simulink model "Drone_BBall_Developer"  (R2020a)
settings: Solver=FixedStepAuto  StartTime=0.0  StopTime=60  FixedStep=.001  RelTol=1e-3
values from neighbouring files (symbols this model uses):
  b = .25*m    (= 0.25)    [Run_Match.m]
  b_ball = .02*m_ball    (= 0.01)    [Run_Match.m]
  b_F_hook = 100    [Run_Match.m]
  b_F_hoop = m_ball * 50    (= 25)    [Run_Match.m]
  b_F_R = m * 20    (= 20)    [Run_Match.m]
  b_F_R_ball = m_ball * 10    (= 5)    [Run_Match.m]
  b_F_R_hook = m_hook * 100    (= 10)    [Run_Match.m]
  B_hook = r_hook^2*6*m_ball*g    (= 0.2943)    [Run_Match.m]
  b_hook = 0.05*m_hook    (= 0.005)    [Run_Match.m]
  b_tether = 1    [Run_Match.m]
  b_th = .1*J    (= 0.0192708333333)    [Run_Match.m]
  b_th_ball = .05*J_ball    (= 0.0009)    [Run_Match.m]
  b_x_net = 80*m_ball*g    (= 392.4)    [Run_Match.m]
  b_y_net = .4*m_ball*g    (= 1.962)    [Run_Match.m]
  drone = struct([])    [Run_Match.m]    (also in animate_drone_bball.m = [-r+w -r-w -r -r r r r+w r-w;             h    h  h  0 0 h  )
  g = 9.81    [Run_Match.m]
  J = 1/4*m*r^2 + 1/12*m*(2*(r+r_M_R))^2    (= 0.192708333333)    [Run_Match.m]
  J_ball = 2/5*m_ball*r_ball^2    (= 0.018)    [Run_Match.m]
  k_f = 4    [Run_Match.m]
  k_F_hook = 10000    [Run_Match.m]
  k_F_hoop = m_ball * 5000    (= 2500)    [Run_Match.m]
  k_F_R = m * 10000    (= 10000)    [Run_Match.m]
  k_F_R_ball = m_ball * 10000    (= 5000)    [Run_Match.m]
  k_F_R_hook = m_hook * 10000    (= 1000)    [Run_Match.m]
  k_tether = 40    [Run_Match.m]
  k_x_net = 200*m_ball*g    (= 981)    [Run_Match.m]
  k_y_net = .5*m_ball*g    (= 2.4525)    [Run_Match.m]
  L_tether = 1.0    (= 1)    [Run_Match.m]
  m = 1    [Run_Match.m]
  m_ball = .5    (= 0.5)    [Run_Match.m]
  m_hook = 0.1*m    (= 0.1)    [Run_Match.m]
  mu_f = .2    (= 0.2)    [Run_Match.m]
  mu_f_gnd = 0.5    [Run_Match.m]
  p_0 = [-5; 5]    [Run_Match.m]
  p_ball_0 = [0; r_ball]    [Run_Match.m]
  p_ball_dot_0 = [0; 12]    [Run_Match.m]
  p_emp = [0; -.4]    [Run_Match.m]
  p_emp_dot = [0; -5]    [Run_Match.m]
  p_hoop = [7.5 8; 8.5 8; -8.5 8; -7.5 8]'    [Run_Match.m]
  p_tether = [0; -0.259]    [Run_Match.m]
  r = 0.5    [Run_Match.m]    (also in animate_drone_bball.m = 0.475)
  r_ball = .3    (= 0.3)    [Run_Match.m]
  r_hook = 0.1    [Run_Match.m]
  r_M_R = 0.25*r    (= 0.125)    [Run_Match.m]
  T_0 = m*g    (= 9.81)    [Run_Match.m]
  T_max = 4*m*g    (= 39.24)    [Run_Match.m]
  T_tau = 0.1    [Run_Match.m]
undefined symbols (not defined in the file or in its folder): clock, M_max, sigbuilder_block, T_aux
libraries: dspswit3 x22, simulink x17, simulink_extras x3, dspmathops x2
(part 2 of 5)

== system Drone_BBall_Developer/Drone 1 Controller/Quadcopter Dynamical Controller ==
  note: Maps the desired net thrust and
      | net moment to the corresponding
      | desired left and right rotor thrust.
  note: Measures the closest
      | angle difference, which
      | may require adding or
      | subtracting 360 degrees.
  note: The upper and lower saturation limits
      | in the X-Axis PID controller limits the
      | maximum desired angle theta to keep
      | the quadcopter upright during flight.
  note: The upper saturation limit in the
      | Y-Axis PID controller leaves some
      | room to impart a moment, even
      | when maximum thrust is desired.
  note: You will almost certainly want the compensator
      | enabled, but temporarily turning it off can be
      | useful during the design process.
  note: By adding an external theta_d to the output
      | of the X-Axis controller, the quadcopter can
      | be made to rotate (e.g., to aim the EMP). I find
      | it works pretty well to implement quick flips this
      | way, and to just fire the EMP whenever the
      |  quadcopter is pointing in the right direction.
  note: Pitch Controller
  note: Y-Axis Controller
  note: X-Axis Controller
  X : Inport
  X_d : Inport  Port=2
  Bypass : ManualSwitch  CurrentSetting=0
  Deg2Rad : Gain  Gain=pi/180
  Demux3 : Demux  Outputs=6
  Demux4 : Demux  Outputs=6
  Diff btwn Angles : Subsystem
  Mux : Mux  Inputs=6
  "Pitch Compensator " : TransferFcn  Numerator=[2 6]  Denominator=[1 10]
  Pitch PID : simulink/Continuous/PID Controller  Controller=PID  Form=Parallel  TimeDomain=Continuous-time  UseExternalTs=off  SampleTime=-1  IntegratorMethod=Forward Euler  FilterMethod=Forward Euler  ControllerParametersSource=internal  P=8  I=0  D=1  UseFilter=on  N=100  TunerSelectOption=Transfer Function Based (PID Tuner App)  InitialConditionSource=internal  InitialConditionForIntegrator=0  InitialConditionForFilter=0  DifferentiatorICPrevScaledInput=0  ExternalReset=none  TrackingMode=off  Kt=1  LimitOutput=off  UpperSaturationLimit=M_max  LowerSaturationLimit=-M_max  LinearizeAsGain=on  AntiWindupMode=none  Kb=1  POutMin=[]  POutMax=[]  IOutMin=[]  IOutMax=[]  DOutMin=[]  DOutMax=[]  NOutMin=[]  NOutMax=[]  SumOutMin=[]  SumOutMax=[]  SaturationOutMin=[]  SaturationOutMax=[]  PParamMin=[]  PParamMax=[]  IParamMin=[]  IParamMax=[]  DParamMin=[]  DParamMax=[]  NParamMin=[]  NParamMax=[]  KbParamMin=[]  KbParamMax=[]  KtParamMin=[]  KtParamMax=[]  KbOutMin=[]  KbOutMax=[]  KtOutMin=[]  KtOutMax=[]  IntegratorOutMin=[]  IntegratorOutMax=[]  FilterOutMin=[]  FilterOutMax=[]  SumI1OutMin=[]  SumI1OutMax=[]  SumI2OutMin=[]  SumI2OutMax=[]  SumI3OutMin=[]  SumI3OutMax=[]  SumI4OutMin=[]  SumI4OutMax=[]  SumDOutMin=[]  SumDOutMax=[]  DifferentiatorOutMin=[]  DifferentiatorOutMax=[]  FilterDiffOutCoefMin=[]  FilterDiffOutCoefMax=[]  ReciprocalOutMin=[]  ReciprocalOutMax=[]  SumDenOutMin=[]  SumDenOutMax=[]  SumNumOutMin=[]  SumNumOutMax=[]  DivideOutMin=[]  DivideOutMax=[]  UdiffTsProdOutMin=[]  UdiffTsProdOutMax=[]  NTsProdOutMin=[]  NTsProdOutMax=[]  UintegralTsProdOutMin=[]  UintegralTsProdOutMax=[]  UngainTsProdOutMin=[]  UngainTsProdOutMax=[]  IntegratorContinuousStateAttributes=''  IntegratorStateMustResolveToSignalObject=off  IntegratorRTWStateStorageClass=Auto  FilterContinuousStateAttributes=''  FilterStateMustResolveToSignalObject=off  FilterRTWStateStorageClass=Auto  ParallelPVariant=InternalParameters  IdealPVariant=Disabled  IVariant=InternalParameters  DVariant=InternalParameters  IntegratorVariant=Continuous  SatVariant=Disabled  AWVariant=Passthrough  PCopyVariant=Disabled  TRVariant=Disabled  FdbkBlocksVariant=Forward  IdealPFdbkVariant=Disabled  SatFdbkVariant=Disabled  DerivativeFilterVariant=ContFilter  NVariant=InternalParameters  NCopyVariant=Disabled  FilterICVariant=InternalICsFilter  IntegratorICVariant=InternalICs  ExternalResetVariant=Disabled  TRSumVariant=Passthrough  SumFdbkVariant=Disabled  SumVariant=Sum_PID  TsampFilterVariant=InternalTs  TsampNgainVariant=Passthrough  TsampIntegralVariant=Passthrough
  Sum : Sum  Inputs=|++
  Sum1 : Sum  Inputs=-|+
  Sum2 : Sum  Inputs=-|+
  Terminator1 : Terminator
  Terminator2 : Terminator
  Terminator7 : Terminator
  Thurst Mapping : Subsystem
  Wrap Angle : Subsystem
  X_Axis PID : simulink/Continuous/PID Controller  Controller=PID  Form=Parallel  TimeDomain=Continuous-time  UseExternalTs=off  SampleTime=-1  IntegratorMethod=Forward Euler  FilterMethod=Forward Euler  ControllerParametersSource=internal  P=8  I=2  D=4  UseFilter=on  N=100  TunerSelectOption=Transfer Function Based (PID Tuner App)  InitialConditionSource=internal  InitialConditionForIntegrator=0  InitialConditionForFilter=0  DifferentiatorICPrevScaledInput=0  ExternalReset=none  TrackingMode=off  Kt=1  LimitOutput=on  UpperSaturationLimit=60  LowerSaturationLimit=-60  LinearizeAsGain=on  AntiWindupMode=clamping  Kb=1  POutMin=[]  POutMax=[]  IOutMin=[]  IOutMax=[]  DOutMin=[]  DOutMax=[]  NOutMin=[]  NOutMax=[]  SumOutMin=[]  SumOutMax=[]  SaturationOutMin=[]  SaturationOutMax=[]  PParamMin=[]  PParamMax=[]  IParamMin=[]  IParamMax=[]  DParamMin=[]  DParamMax=[]  NParamMin=[]  NParamMax=[]  KbParamMin=[]  KbParamMax=[]  KtParamMin=[]  KtParamMax=[]  KbOutMin=[]  KbOutMax=[]  KtOutMin=[]  KtOutMax=[]  IntegratorOutMin=[]  IntegratorOutMax=[]  FilterOutMin=[]  FilterOutMax=[]  SumI1OutMin=[]  SumI1OutMax=[]  SumI2OutMin=[]  SumI2OutMax=[]  SumI3OutMin=[]  SumI3OutMax=[]  SumI4OutMin=[]  SumI4OutMax=[]  SumDOutMin=[]  SumDOutMax=[]  DifferentiatorOutMin=[]  DifferentiatorOutMax=[]  FilterDiffOutCoefMin=[]  FilterDiffOutCoefMax=[]  ReciprocalOutMin=[]  ReciprocalOutMax=[]  SumDenOutMin=[]  SumDenOutMax=[]  SumNumOutMin=[]  SumNumOutMax=[]  DivideOutMin=[]  DivideOutMax=[]  UdiffTsProdOutMin=[]  UdiffTsProdOutMax=[]  NTsProdOutMin=[]  NTsProdOutMax=[]  UintegralTsProdOutMin=[]  UintegralTsProdOutMax=[]  UngainTsProdOutMin=[]  UngainTsProdOutMax=[]  IntegratorContinuousStateAttributes=''  IntegratorStateMustResolveToSignalObject=off  IntegratorRTWStateStorageClass=Auto  FilterContinuousStateAttributes=''  FilterStateMustResolveToSignalObject=off  FilterRTWStateStorageClass=Auto  ParallelPVariant=InternalParameters  IdealPVariant=Disabled  IVariant=InternalParameters  DVariant=InternalParameters  IntegratorVariant=Continuous  SatVariant=Enabled  AWVariant=ContClampingParallel  PCopyVariant=Disabled  TRVariant=Disabled  FdbkBlocksVariant=Forward  IdealPFdbkVariant=Disabled  SatFdbkVariant=Disabled  DerivativeFilterVariant=ContFilter  NVariant=InternalParameters  NCopyVariant=Disabled  FilterICVariant=InternalICsFilter  IntegratorICVariant=InternalICs  ExternalResetVariant=Disabled  TRSumVariant=Passthrough  SumFdbkVariant=Disabled  SumVariant=Sum_PID  TsampFilterVariant=InternalTs  TsampNgainVariant=Passthrough  TsampIntegralVariant=Passthrough
  Y_Axis PID : simulink/Continuous/PID Controller  Controller=PID  Form=Parallel  TimeDomain=Continuous-time  UseExternalTs=off  SampleTime=-1  IntegratorMethod=Forward Euler  FilterMethod=Forward Euler  ControllerParametersSource=internal  P=36.8701654473811  I=116.471336399404  D=12.6703199505361  UseFilter=on  N=100  TunerSelectOption=Transfer Function Based (PID Tuner App)  InitialConditionSource=internal  InitialConditionForIntegrator=m*g  InitialConditionForFilter=0  DifferentiatorICPrevScaledInput=0  ExternalReset=none  TrackingMode=off  Kt=1  LimitOutput=on  UpperSaturationLimit=T_max - 2*T_aux  LowerSaturationLimit=0  LinearizeAsGain=on  AntiWindupMode=clamping  Kb=1  POutMin=[]  POutMax=[]  IOutMin=[]  IOutMax=[]  DOutMin=[]  DOutMax=[]  NOutMin=[]  NOutMax=[]  SumOutMin=[]  SumOutMax=[]  SaturationOutMin=[]  SaturationOutMax=[]  PParamMin=[]  PParamMax=[]  IParamMin=[]  IParamMax=[]  DParamMin=[]  DParamMax=[]  NParamMin=[]  NParamMax=[]  KbParamMin=[]  KbParamMax=[]  KtParamMin=[]  KtParamMax=[]  KbOutMin=[]  KbOutMax=[]  KtOutMin=[]  KtOutMax=[]  IntegratorOutMin=[]  IntegratorOutMax=[]  FilterOutMin=[]  FilterOutMax=[]  SumI1OutMin=[]  SumI1OutMax=[]  SumI2OutMin=[]  SumI2OutMax=[]  SumI3OutMin=[]  SumI3OutMax=[]  SumI4OutMin=[]  SumI4OutMax=[]  SumDOutMin=[]  SumDOutMax=[]  DifferentiatorOutMin=[]  DifferentiatorOutMax=[]  FilterDiffOutCoefMin=[]  FilterDiffOutCoefMax=[]  ReciprocalOutMin=[]  ReciprocalOutMax=[]  SumDenOutMin=[]  SumDenOutMax=[]  SumNumOutMin=[]  SumNumOutMax=[]  DivideOutMin=[]  DivideOutMax=[]  UdiffTsProdOutMin=[]  UdiffTsProdOutMax=[]  NTsProdOutMin=[]  NTsProdOutMax=[]  UintegralTsProdOutMin=[]  UintegralTsProdOutMax=[]  UngainTsProdOutMin=[]  UngainTsProdOutMax=[]  IntegratorContinuousStateAttributes=''  IntegratorStateMustResolveToSignalObject=off  IntegratorRTWStateStorageClass=Auto  FilterContinuousStateAttributes=''  FilterStateMustResolveToSignalObject=off  FilterRTWStateStorageClass=Auto  ParallelPVariant=InternalParameters  IdealPVariant=Disabled  IVariant=InternalParameters  DVariant=InternalParameters  IntegratorVariant=Continuous  SatVariant=Enabled  AWVariant=ContClampingParallel  PCopyVariant=Disabled  TRVariant=Disabled  FdbkBlocksVariant=Forward  IdealPFdbkVariant=Disabled  SatFdbkVariant=Disabled  DerivativeFilterVariant=ContFilter  NVariant=InternalParameters  NCopyVariant=Disabled  FilterICVariant=InternalICsFilter  IntegratorICVariant=InternalICs  ExternalResetVariant=Disabled  TRSumVariant=Passthrough  SumFdbkVariant=Disabled  SumVariant=Sum_PID  TsampFilterVariant=InternalTs  TsampNgainVariant=Passthrough  TsampIntegralVariant=Passthrough
  T_L_d : Outport  VectorParamsAs1DForOutWhenUnconnected=off
  T_R_d : Outport  Port=2  VectorParamsAs1DForOutWhenUnconnected=off
  X_d_adj : Outport  Port=3  VectorParamsAs1DForOutWhenUnconnected=off
  wires:
  Thurst Mapping/2(T_R_d) -> T_R_d/1
  X_Axis PID/1 -> Deg2Rad/1
  "Pitch Compensator "/1 -> Bypass/2
  Bypass/1 -> Pitch PID/1
  Pitch PID/1 -> Thurst Mapping/1(M_d)
  Thurst Mapping/1(T_L_d) -> T_L_d/1
  Y_Axis PID/1 -> Thurst Mapping/2(T_d)
  Demux3/6 -> Mux/6
  Demux4/6 -> Terminator7/1
  Demux4/5 -> Diff btwn Angles/1(theta)  "theta"
  X_d/1 -> Demux3/1
  Demux4/1 -> Sum1/1  "x"
  Demux3/1 -> Mux/1, Sum1/2  "x_d"
  Demux4/3 -> Sum2/1  "y"
  Demux3/3 -> Sum2/2, Mux/3  "y_d"
  Demux3/2 -> Mux/2
  Demux3/4 -> Mux/4
  Demux3/5 -> Sum/2
  Sum/1 -> Wrap Angle/1(raw), Diff btwn Angles/2(theta_d)  "theta_d"
  X/1 -> Demux4/1
  Mux/1 -> X_d_adj/1
  Diff btwn Angles/1(e) -> Bypass/1, "Pitch Compensator "/1
  Wrap Angle/1(wrap) -> Mux/5
  Demux4/2 -> Terminator1/1
  Demux4/4 -> Terminator2/1
  Sum2/1 -> Y_Axis PID/1
  Sum1/1 -> X_Axis PID/1
  Deg2Rad/1 -> Sum/1

== system Drone_BBall_Developer/Drone 1 Controller/Quadcopter Dynamical Controller (Arena Frame) ==
  note: Maps the desired net thrust and
      | net moment to the corresponding
      | desired left and right rotor thrust.
  note: Measures the closest
      | angle difference, which
      | may require adding or
      | subtracting 360 degrees.
  note: The upper and lower saturation limits
      | in the X-Axis PID controller limits the
      | maximum desired angle theta to keep
      | the quadcopter upright during flight.
  note: The upper saturation limit in the
      | Y-Axis PID controller leaves some
      | room to impart a moment, even
      | when maximum thrust is desired.
  note: You will almost certainly want the compensator
      | enabled, but temporarily turning it off can be
      | useful during the design process.
  note: By adding an external theta_d to the output
      | of the X-Axis controller, the quadcopter can
      | be made to rotate (e.g., to aim the EMP). I find
      | it works pretty well to implement quick flips this
      | way, and to just fire the EMP whenever the
      |  quadcopter is pointing in the right direction.
  note: Pitch Controller
  note: Y-Axis Controller
  note: X-Axis Controller
  X : Inport
  X_d : Inport  Port=2
  Bypass : ManualSwitch
  Deg2Rad : Gain  Gain=pi/180
  Demux3 : Demux  Outputs=6
  Demux4 : Demux  Outputs=6
  Diff btwn Angles : Subsystem
  Mux : Mux  Inputs=6
  "Pitch Compensator " : TransferFcn  Numerator=[2 6]  Denominator=[1 10]
  Pitch PID : simulink/Continuous/PID Controller  Controller=PID  Form=Parallel  TimeDomain=Continuous-time  UseExternalTs=off  SampleTime=-1  IntegratorMethod=Forward Euler  FilterMethod=Forward Euler  ControllerParametersSource=internal  P=8  I=0  D=1  UseFilter=on  N=100  TunerSelectOption=Transfer Function Based (PID Tuner App)  InitialConditionSource=internal  InitialConditionForIntegrator=0  InitialConditionForFilter=0  DifferentiatorICPrevScaledInput=0  ExternalReset=none  TrackingMode=off  Kt=1  LimitOutput=off  UpperSaturationLimit=M_max  LowerSaturationLimit=-M_max  LinearizeAsGain=on  AntiWindupMode=none  Kb=1  POutMin=[]  POutMax=[]  IOutMin=[]  IOutMax=[]  DOutMin=[]  DOutMax=[]  NOutMin=[]  NOutMax=[]  SumOutMin=[]  SumOutMax=[]  SaturationOutMin=[]  SaturationOutMax=[]  PParamMin=[]  PParamMax=[]  IParamMin=[]  IParamMax=[]  DParamMin=[]  DParamMax=[]  NParamMin=[]  NParamMax=[]  KbParamMin=[]  KbParamMax=[]  KtParamMin=[]  KtParamMax=[]  KbOutMin=[]  KbOutMax=[]  KtOutMin=[]  KtOutMax=[]  IntegratorOutMin=[]  IntegratorOutMax=[]  FilterOutMin=[]  FilterOutMax=[]  SumI1OutMin=[]  SumI1OutMax=[]  SumI2OutMin=[]  SumI2OutMax=[]  SumI3OutMin=[]  SumI3OutMax=[]  SumI4OutMin=[]  SumI4OutMax=[]  SumDOutMin=[]  SumDOutMax=[]  DifferentiatorOutMin=[]  DifferentiatorOutMax=[]  FilterDiffOutCoefMin=[]  FilterDiffOutCoefMax=[]  ReciprocalOutMin=[]  ReciprocalOutMax=[]  SumDenOutMin=[]  SumDenOutMax=[]  SumNumOutMin=[]  SumNumOutMax=[]  DivideOutMin=[]  DivideOutMax=[]  UdiffTsProdOutMin=[]  UdiffTsProdOutMax=[]  NTsProdOutMin=[]  NTsProdOutMax=[]  UintegralTsProdOutMin=[]  UintegralTsProdOutMax=[]  UngainTsProdOutMin=[]  UngainTsProdOutMax=[]  IntegratorContinuousStateAttributes=''  IntegratorStateMustResolveToSignalObject=off  IntegratorRTWStateStorageClass=Auto  FilterContinuousStateAttributes=''  FilterStateMustResolveToSignalObject=off  FilterRTWStateStorageClass=Auto  ParallelPVariant=InternalParameters  IdealPVariant=Disabled  IVariant=InternalParameters  DVariant=InternalParameters  IntegratorVariant=Continuous  SatVariant=Disabled  AWVariant=Passthrough  PCopyVariant=Disabled  TRVariant=Disabled  FdbkBlocksVariant=Forward  IdealPFdbkVariant=Disabled  SatFdbkVariant=Disabled  DerivativeFilterVariant=ContFilter  NVariant=InternalParameters  NCopyVariant=Disabled  FilterICVariant=InternalICsFilter  IntegratorICVariant=InternalICs  ExternalResetVariant=Disabled  TRSumVariant=Passthrough  SumFdbkVariant=Disabled  SumVariant=Sum_PID  TsampFilterVariant=InternalTs  TsampNgainVariant=Passthrough  TsampIntegralVariant=Passthrough
  Sum : Sum  Inputs=|++
  Sum1 : Sum  Inputs=-|+
  Sum2 : Sum  Inputs=-|+
  Terminator1 : Terminator
  Terminator2 : Terminator
  Terminator7 : Terminator
  Thurst Mapping : Subsystem
  Wrap Angle : Subsystem
  X_Axis PID : simulink/Continuous/PID Controller  Controller=PID  Form=Parallel  TimeDomain=Continuous-time  UseExternalTs=off  SampleTime=-1  IntegratorMethod=Forward Euler  FilterMethod=Forward Euler  ControllerParametersSource=internal  P=8  I=2  D=4  UseFilter=on  N=100  TunerSelectOption=Transfer Function Based (PID Tuner App)  InitialConditionSource=internal  InitialConditionForIntegrator=0  InitialConditionForFilter=0  DifferentiatorICPrevScaledInput=0  ExternalReset=none  TrackingMode=off  Kt=1  LimitOutput=on  UpperSaturationLimit=60  LowerSaturationLimit=-60  LinearizeAsGain=on  AntiWindupMode=clamping  Kb=1  POutMin=[]  POutMax=[]  IOutMin=[]  IOutMax=[]  DOutMin=[]  DOutMax=[]  NOutMin=[]  NOutMax=[]  SumOutMin=[]  SumOutMax=[]  SaturationOutMin=[]  SaturationOutMax=[]  PParamMin=[]  PParamMax=[]  IParamMin=[]  IParamMax=[]  DParamMin=[]  DParamMax=[]  NParamMin=[]  NParamMax=[]  KbParamMin=[]  KbParamMax=[]  KtParamMin=[]  KtParamMax=[]  KbOutMin=[]  KbOutMax=[]  KtOutMin=[]  KtOutMax=[]  IntegratorOutMin=[]  IntegratorOutMax=[]  FilterOutMin=[]  FilterOutMax=[]  SumI1OutMin=[]  SumI1OutMax=[]  SumI2OutMin=[]  SumI2OutMax=[]  SumI3OutMin=[]  SumI3OutMax=[]  SumI4OutMin=[]  SumI4OutMax=[]  SumDOutMin=[]  SumDOutMax=[]  DifferentiatorOutMin=[]  DifferentiatorOutMax=[]  FilterDiffOutCoefMin=[]  FilterDiffOutCoefMax=[]  ReciprocalOutMin=[]  ReciprocalOutMax=[]  SumDenOutMin=[]  SumDenOutMax=[]  SumNumOutMin=[]  SumNumOutMax=[]  DivideOutMin=[]  DivideOutMax=[]  UdiffTsProdOutMin=[]  UdiffTsProdOutMax=[]  NTsProdOutMin=[]  NTsProdOutMax=[]  UintegralTsProdOutMin=[]  UintegralTsProdOutMax=[]  UngainTsProdOutMin=[]  UngainTsProdOutMax=[]  IntegratorContinuousStateAttributes=''  IntegratorStateMustResolveToSignalObject=off  IntegratorRTWStateStorageClass=Auto  FilterContinuousStateAttributes=''  FilterStateMustResolveToSignalObject=off  FilterRTWStateStorageClass=Auto  ParallelPVariant=InternalParameters  IdealPVariant=Disabled  IVariant=InternalParameters  DVariant=InternalParameters  IntegratorVariant=Continuous  SatVariant=Enabled  AWVariant=ContClampingParallel  PCopyVariant=Disabled  TRVariant=Disabled  FdbkBlocksVariant=Forward  IdealPFdbkVariant=Disabled  SatFdbkVariant=Disabled  DerivativeFilterVariant=ContFilter  NVariant=InternalParameters  NCopyVariant=Disabled  FilterICVariant=InternalICsFilter  IntegratorICVariant=InternalICs  ExternalResetVariant=Disabled  TRSumVariant=Passthrough  SumFdbkVariant=Disabled  SumVariant=Sum_PID  TsampFilterVariant=InternalTs  TsampNgainVariant=Passthrough  TsampIntegralVariant=Passthrough
  Y_Axis PID : simulink/Continuous/PID Controller  Controller=PID  Form=Parallel  TimeDomain=Continuous-time  UseExternalTs=off  SampleTime=-1  IntegratorMethod=Forward Euler  FilterMethod=Forward Euler  ControllerParametersSource=internal  P=5  I=4  D=1  UseFilter=on  N=100  TunerSelectOption=Transfer Function Based (PID Tuner App)  InitialConditionSource=internal  InitialConditionForIntegrator=m*g  InitialConditionForFilter=0  DifferentiatorICPrevScaledInput=0  ExternalReset=none  TrackingMode=off  Kt=1  LimitOutput=on  UpperSaturationLimit=T_max - 0.2  LowerSaturationLimit=0  LinearizeAsGain=on  AntiWindupMode=clamping  Kb=1  POutMin=[]  POutMax=[]  IOutMin=[]  IOutMax=[]  DOutMin=[]  DOutMax=[]  NOutMin=[]  NOutMax=[]  SumOutMin=[]  SumOutMax=[]  SaturationOutMin=[]  SaturationOutMax=[]  PParamMin=[]  PParamMax=[]  IParamMin=[]  IParamMax=[]  DParamMin=[]  DParamMax=[]  NParamMin=[]  NParamMax=[]  KbParamMin=[]  KbParamMax=[]  KtParamMin=[]  KtParamMax=[]  KbOutMin=[]  KbOutMax=[]  KtOutMin=[]  KtOutMax=[]  IntegratorOutMin=[]  IntegratorOutMax=[]  FilterOutMin=[]  FilterOutMax=[]  SumI1OutMin=[]  SumI1OutMax=[]  SumI2OutMin=[]  SumI2OutMax=[]  SumI3OutMin=[]  SumI3OutMax=[]  SumI4OutMin=[]  SumI4OutMax=[]  SumDOutMin=[]  SumDOutMax=[]  DifferentiatorOutMin=[]  DifferentiatorOutMax=[]  FilterDiffOutCoefMin=[]  FilterDiffOutCoefMax=[]  ReciprocalOutMin=[]  ReciprocalOutMax=[]  SumDenOutMin=[]  SumDenOutMax=[]  SumNumOutMin=[]  SumNumOutMax=[]  DivideOutMin=[]  DivideOutMax=[]  UdiffTsProdOutMin=[]  UdiffTsProdOutMax=[]  NTsProdOutMin=[]  NTsProdOutMax=[]  UintegralTsProdOutMin=[]  UintegralTsProdOutMax=[]  UngainTsProdOutMin=[]  UngainTsProdOutMax=[]  IntegratorContinuousStateAttributes=''  IntegratorStateMustResolveToSignalObject=off  IntegratorRTWStateStorageClass=Auto  FilterContinuousStateAttributes=''  FilterStateMustResolveToSignalObject=off  FilterRTWStateStorageClass=Auto  ParallelPVariant=InternalParameters  IdealPVariant=Disabled  IVariant=InternalParameters  DVariant=InternalParameters  IntegratorVariant=Continuous  SatVariant=Enabled  AWVariant=ContClampingParallel  PCopyVariant=Disabled  TRVariant=Disabled  FdbkBlocksVariant=Forward  IdealPFdbkVariant=Disabled  SatFdbkVariant=Disabled  DerivativeFilterVariant=ContFilter  NVariant=InternalParameters  NCopyVariant=Disabled  FilterICVariant=InternalICsFilter  IntegratorICVariant=InternalICs  ExternalResetVariant=Disabled  TRSumVariant=Passthrough  SumFdbkVariant=Disabled  SumVariant=Sum_PID  TsampFilterVariant=InternalTs  TsampNgainVariant=Passthrough  TsampIntegralVariant=Passthrough
  T_L_d : Outport  VectorParamsAs1DForOutWhenUnconnected=off
  T_R_d : Outport  Port=2  VectorParamsAs1DForOutWhenUnconnected=off
  X_d_adj : Outport  Port=3  VectorParamsAs1DForOutWhenUnconnected=off
  wires:
  Thurst Mapping/2(T_R_d) -> T_R_d/1
  X_Axis PID/1 -> Deg2Rad/1
  "Pitch Compensator "/1 -> Bypass/2
  Bypass/1 -> Pitch PID/1
  Pitch PID/1 -> Thurst Mapping/1(M_d)
  Thurst Mapping/1(T_L_d) -> T_L_d/1
  Y_Axis PID/1 -> Thurst Mapping/2(T_d)
  Demux3/6 -> Mux/6
  Demux4/6 -> Terminator7/1
  Demux4/5 -> Diff btwn Angles/1(theta)  "theta"
  X_d/1 -> Demux3/1
  Demux4/1 -> Sum1/1  "x"
  Demux3/1 -> Mux/1, Sum1/2  "x_d"
  Demux4/3 -> Sum2/1  "y"
  Demux3/3 -> Sum2/2, Mux/3  "y_d"
  Demux3/2 -> Mux/2
  Demux3/4 -> Mux/4
  Demux3/5 -> Sum/2
  Sum/1 -> Wrap Angle/1(raw), Diff btwn Angles/2(theta_d)  "theta_d"
  X/1 -> Demux4/1
  Mux/1 -> X_d_adj/1
  Diff btwn Angles/1(e) -> Bypass/1, "Pitch Compensator "/1
  Wrap Angle/1(wrap) -> Mux/5
  Demux4/2 -> Terminator1/1
  Demux4/4 -> Terminator2/1
  Sum2/1 -> Y_Axis PID/1
  Sum1/1 -> X_Axis PID/1
  Deg2Rad/1 -> Sum/1

== system Drone_BBall_Developer/Drone 1 Controller/Quadcopter Dynamical Controller (Drone Frame) ==
  note: Maps the desired net thrust and
      | net moment to the corresponding
      | desired left and right rotor thrust.
  note: Measures the closest
      | angle difference, which
      | may require adding or
      | subtracting 360 degrees.
  note: These subsystems rotate the error
      | signal, and its derivative, so that they
      | are reported in the quadcopter's
      | frame of reference. This prevents its
      | rotation from affecting the derivative
      | error terms used by the PID controllers.
  note: The upper and lower saturation limits
      | in the X-Axis PID controller limits the
      | maximum desired angle theta to keep
      | the quadcopter upright during flight.
      |
      | (I had to build custom anti-windup
      | PID controllers for X- and Y-axis to
      | separate e and e_dot inputs.)
  note: The upper saturation limit in the
      | Y-Axis PID controller leaves some
      | room to impart a moment, even
      | when maximum thrust is desired.
  note: You will almost certainly want the compensator
      | enabled, but temporarily turning it off can be
      | useful during the design process.
  note: By adding an external theta_d to the output of the X-Axis controller,
      | the quadcopter can be made to rotate (e.g., to aim the EMP). I find
      | it works pretty well to implement quick flips this way, and to just fire
      | the EMP whenever the quadcopter is pointing in the right direction.
  note: Pitch Controller
  note: Y-Axis Controller
  note: X-Axis Controller
  note: Rotate Error Signals
  X : Inport
  X_d : Inport  Port=2
  Bypass : ManualSwitch  CurrentSetting=0
  Demux : Demux  Outputs=2
  Demux1 : Demux  Outputs=2
  Demux3 : Demux  Outputs=6
  Demux4 : Demux  Outputs=6
  Diff btwn Angles : Subsystem
  Mux : Mux  Inputs=6
  Mux1 : Mux  Inputs=2
  Mux3 : Mux  Inputs=2
  "Pitch Compensator " : TransferFcn  Numerator=[2 6]  Denominator=[1 10]
  Pitch PID : simulink/Continuous/PID Controller  Controller=PID  Form=Parallel  TimeDomain=Continuous-time  UseExternalTs=off  SampleTime=-1  IntegratorMethod=Forward Euler  FilterMethod=Forward Euler  ControllerParametersSource=internal  P=8  I=0  D=1  UseFilter=on  N=100  TunerSelectOption=Transfer Function Based (PID Tuner App)  InitialConditionSource=internal  InitialConditionForIntegrator=0  InitialConditionForFilter=0  DifferentiatorICPrevScaledInput=0  ExternalReset=none  TrackingMode=off  Kt=1  LimitOutput=off  UpperSaturationLimit=M_max  LowerSaturationLimit=-M_max  LinearizeAsGain=on  AntiWindupMode=none  Kb=1  POutMin=[]  POutMax=[]  IOutMin=[]  IOutMax=[]  DOutMin=[]  DOutMax=[]  NOutMin=[]  NOutMax=[]  SumOutMin=[]  SumOutMax=[]  SaturationOutMin=[]  SaturationOutMax=[]  PParamMin=[]  PParamMax=[]  IParamMin=[]  IParamMax=[]  DParamMin=[]  DParamMax=[]  NParamMin=[]  NParamMax=[]  KbParamMin=[]  KbParamMax=[]  KtParamMin=[]  KtParamMax=[]  KbOutMin=[]  KbOutMax=[]  KtOutMin=[]  KtOutMax=[]  IntegratorOutMin=[]  IntegratorOutMax=[]  FilterOutMin=[]  FilterOutMax=[]  SumI1OutMin=[]  SumI1OutMax=[]  SumI2OutMin=[]  SumI2OutMax=[]  SumI3OutMin=[]  SumI3OutMax=[]  SumI4OutMin=[]  SumI4OutMax=[]  SumDOutMin=[]  SumDOutMax=[]  DifferentiatorOutMin=[]  DifferentiatorOutMax=[]  FilterDiffOutCoefMin=[]  FilterDiffOutCoefMax=[]  ReciprocalOutMin=[]  ReciprocalOutMax=[]  SumDenOutMin=[]  SumDenOutMax=[]  SumNumOutMin=[]  SumNumOutMax=[]  DivideOutMin=[]  DivideOutMax=[]  UdiffTsProdOutMin=[]  UdiffTsProdOutMax=[]  NTsProdOutMin=[]  NTsProdOutMax=[]  UintegralTsProdOutMin=[]  UintegralTsProdOutMax=[]  UngainTsProdOutMin=[]  UngainTsProdOutMax=[]  IntegratorContinuousStateAttributes=''  IntegratorStateMustResolveToSignalObject=off  IntegratorRTWStateStorageClass=Auto  FilterContinuousStateAttributes=''  FilterStateMustResolveToSignalObject=off  FilterRTWStateStorageClass=Auto  ParallelPVariant=InternalParameters  IdealPVariant=Disabled  IVariant=InternalParameters  DVariant=InternalParameters  IntegratorVariant=Continuous  SatVariant=Disabled  AWVariant=Passthrough  PCopyVariant=Disabled  TRVariant=Disabled  FdbkBlocksVariant=Forward  IdealPFdbkVariant=Disabled  SatFdbkVariant=Disabled  DerivativeFilterVariant=ContFilter  NVariant=InternalParameters  NCopyVariant=Disabled  FilterICVariant=InternalICsFilter  IntegratorICVariant=InternalICs  ExternalResetVariant=Disabled  TRSumVariant=Passthrough  SumFdbkVariant=Disabled  SumVariant=Sum_PID  TsampFilterVariant=InternalTs  TsampNgainVariant=Passthrough  TsampIntegralVariant=Passthrough
  Rotate e (CCW) : Subsystem
  Rotate e_dot (CCW) : Subsystem
  Sum : Sum  Inputs=|++
  Sum{1..4} (4 alike) : Sum  Inputs=-|+
  Terminator7 : Terminator
  Thurst Mapping : Subsystem
  Wrap Angle : Subsystem
  X-Axis PID : Subsystem  mask{u_max=40, K_P=8, K_I=2, K_D=4}
      mask prompts: u_max "Integration Bound (degrees)"; K_P "Proportional Gain"; K_I "Integral Gain"; K_D "Derivative Gain"
  Y-Axis PID : Subsystem  mask{u_max=T_max - 0.2, u_0=m*g, K_P=5, K_I=4, K_D=1}
      mask prompts: u_max "Integration Bound (N)"; u_0 "Initial Thrust (N)"; K_P "Proportional Gain"; K_I "Integral Gain"; K_D "Derivative Gain"
  T_L_d : Outport  VectorParamsAs1DForOutWhenUnconnected=off
  T_R_d : Outport  Port=2  VectorParamsAs1DForOutWhenUnconnected=off
  X_d_adj : Outport  Port=3  VectorParamsAs1DForOutWhenUnconnected=off
  wires:
  Thurst Mapping/2(T_R_d) -> T_R_d/1
  X-Axis PID/1(u) -> Sum/1
  "Pitch Compensator "/1 -> Bypass/2
  Bypass/1 -> Pitch PID/1
  Pitch PID/1 -> Thurst Mapping/1(M_d)
  Thurst Mapping/1(T_L_d) -> T_L_d/1
  Rotate e_dot (CCW)/1(R(theta)*p) -> Demux1/1
  Rotate e (CCW)/1(R(theta)*p) -> Demux/1
  Demux1/1 -> X-Axis PID/2(e_dot)
  Demux1/2 -> Y-Axis PID/2(e_dot)
  Y-Axis PID/1(u) -> Thurst Mapping/2(T_d)
  Demux3/6 -> Mux/6
  Demux4/6 -> Terminator7/1
  Demux4/5 -> Rotate e (CCW)/2(theta), Rotate e_dot (CCW)/2(theta), Diff btwn Angles/1(theta)  "theta"
  Mux1/1 -> Rotate e (CCW)/1(p)
  Mux3/1 -> Rotate e_dot (CCW)/1(p)
  X_d/1 -> Demux3/1
  Demux4/1 -> Sum1/1  "x"
  Demux3/1 -> Mux/1, Sum1/2  "x_d"
  Sum1/1 -> Mux1/1
  Demux4/3 -> Sum2/1  "y"
  Demux3/3 -> Mux/3, Sum2/2  "y_d"
  Demux3/2 -> Mux/2, Sum3/2
  Demux4/2 -> Sum3/1
  Sum3/1 -> Mux3/1
  Sum4/1 -> Mux3/2
  Demux4/4 -> Sum4/1
  Demux3/4 -> Mux/4, Sum4/2
  Demux3/5 -> Sum/2
  Sum/1 -> Wrap Angle/1(raw), Diff btwn Angles/2(theta_d)  "theta_d"
  X/1 -> Demux4/1
  Mux/1 -> X_d_adj/1
  Diff btwn Angles/1(e) -> Bypass/1, "Pitch Compensator "/1
  Wrap Angle/1(wrap) -> Mux/5
  Demux/1 -> X-Axis PID/1(e)
  Sum2/1 -> Mux1/2
  Demux/2 -> Y-Axis PID/1(e)

== system Drone_BBall_Developer/Drone 1 Controller/Reference Inputs for Testing ==
  Demux : Demux  Tag=STV Demux  Outputs=5
      settings: DisplayOption=none
  FromWs : FromWorkspace  Tag=STV FromWs  VariableName=tuvar
      SigBuilderData=|
      | common.afterFinalStr = 'Extrapolate'
      | common.sampleTime = 0
      | dataSet.timeRange = [0 20]
      | dataSet.name = 'Reference Trajectory'
      | sbobj.Groups.Name = 'Reference Trajectory'
      | sbobj.Groups.Signals(1).Name = 'x_d'
      | sbobj.Groups.Signals(1).XData = [0 4 5 9 10 14 20]
      | sbobj.Groups.Signals(1).YData = [-5 5 5 -5 -5 5 5]
      | sbobj.Groups.Signals(2).Name = 'y_d'
      | sbobj.Groups.Signals(2).XData = [0 3 6 8 11 13 16 20]
      | sbobj.Groups.Signals(2).YData = [5 5 10 10 5 5 10 10]
      | sbobj.Groups.Signals(3).Name = 'theta_d'
      | sbobj.Groups.Signals(3).XData = [0 5 5.5 20]
      | sbobj.Groups.Signals(3).YData = [0 0 360 360]
      | sbobj.Groups.Signals(4).Name = 'fire_emp'
      | sbobj.Groups.Signals(4).XData = [0 4 4.5 4.5 5 5 5.5 7 7 7.5 7.5 8 8 11 11 12 12 12.9 12.9 20]
      | sbobj.Groups.Signals(4).YData = [0 0 0 1 1 0 0 0 1 1 0 0 1 1 0 0 1 1 0 0]
      | sbobj.Groups.Signals(5).Name = 'mag_on'
      | sbobj.Groups.Signals(5).XData = [0 12 12 20]
      | sbobj.Groups.Signals(5).YData = [1 1 0 0]
      | sbobj.Groups.TimeRange = [0 20]
  x_d : Outport  Tag=STV Outport  VectorParamsAs1DForOutWhenUnconnected=off
  y_d : Outport  Tag=STV Outport  Port=2  VectorParamsAs1DForOutWhenUnconnected=off
  theta_d : Outport  Tag=STV Outport  Port=3
  fire_emp : Outport  Tag=STV Outport  Port=4  VectorParamsAs1DForOutWhenUnconnected=off
  mag_on : Outport  Tag=STV Outport  Port=5  VectorParamsAs1DForOutWhenUnconnected=off
  wires:
  FromWs/1 -> Demux/1
  Demux/1 -> x_d/1
  Demux/2 -> y_d/1
  Demux/3 -> theta_d/1
  Demux/4 -> fire_emp/1
  Demux/5 -> mag_on/1

== system Drone_BBall_Developer/Drone 1 Controller/Useful Scopes for Troubleshooting ==
  X : Inport
  X_d : Inport  Port=2
  Demux1 : Demux  Outputs=6
  Demux2 : Demux  Outputs=6
  Drone Kinematics : Scope  NumInputPorts=6
  Gain1 : Gain  Gain=180/pi
  Gain2 : Gain  Gain=180/pi
  Individual Scopes : Scope  NumInputPorts=2
  Terminator{1..6} (6 alike) : Terminator
  x : Scope  NumInputPorts=2
  y : Scope  NumInputPorts=2
  wires:
  Demux2/1 -> x/2, Drone Kinematics/2  "x_d(t)"
  Demux2/3 -> y/2, Drone Kinematics/4  "y_d(t)"
  Demux1/4 -> Terminator4/1
  Gain2/1 -> Individual Scopes/1  "theta (deg)"
  Demux1/5 -> Drone Kinematics/5, Gain2/1  "theta(t)"
  Demux1/2 -> Terminator3/1
  Demux1/1 -> x/1, Drone Kinematics/1  "x(t)"
  Demux1/3 -> y/1, Drone Kinematics/3  "y(t)"
  Demux1/6 -> Terminator5/1
  Demux2/5 -> Gain1/1, Drone Kinematics/6  "theta_d(t)"
  Gain1/1 -> Individual Scopes/2  "theta_d (deg)"
  X/1 -> Demux1/1
  X_d/1 -> Demux2/1
  Demux2/4 -> Terminator2/1
  Demux2/6 -> Terminator6/1
  Demux2/2 -> Terminator1/1

== system Drone_BBall_Developer/Drone 1 Dynamics/Hook Plant ==
  mag_on : Inport
  X_ball : Inport  Port=2
  X_drone : Inport  Port=3
  Constant : Constant  Value=0
  Constant1 : Constant  Value=[0; -m_hook*g]
  Demux{,1..3} (4 alike) : Demux  Outputs=2
  Gain : Gain  Gain=-1
  Ground Reactions : Subsystem
  Hook Dynamics : Subsystem
  Linear Dynamics : Subsystem
  Mux : Mux  Inputs=3
  Mux1 : Mux  Inputs=6
  Mux3 : Mux  Inputs=3
  Sum : Sum  Inputs=+|+-+
  Tether Dynamics : Subsystem
  X_hook : Outport  VectorParamsAs1DForOutWhenUnconnected=off
  FM_ball : Outport  Port=2  VectorParamsAs1DForOutWhenUnconnected=off
  F_tether_r : Outport  Port=3  VectorParamsAs1DForOutWhenUnconnected=off
  FM_tether_rxn : Outport  Port=4  VectorParamsAs1DForOutWhenUnconnected=off
  wires:
  Constant/1 -> Mux1/6, Mux1/5
  Demux2/1 -> Mux1/2  "x_dot"
  Demux1/2 -> Mux1/3  "y"
  Demux1/1 -> Mux1/1  "x"
  Linear Dynamics/2(p_dot) -> Demux2/1  "p_dot"
  Demux2/2 -> Mux1/4  "y_dot"
  Linear Dynamics/1(p) -> Demux1/1  "p"
  Constant1/1 -> Sum/1
  Ground Reactions/1(F_R) -> Sum/2
  Sum/1 -> Linear Dynamics/1(F)
  mag_on/1 -> Hook Dynamics/3(mag_on)
  Mux1/1 -> X_hook/1, Ground Reactions/1(X), Tether Dynamics/2(X_hook), Hook Dynamics/1(X_hook)
  X_ball/1 -> Hook Dynamics/2(X_ball)
  Hook Dynamics/1(F_ball) -> Sum/3, Demux/1
  Hook Dynamics/2(M_ball) -> Mux/3
  Mux/1 -> FM_ball/1
  Demux/1 -> Mux/1
  Demux/2 -> Mux/2
  Demux3/2 -> Mux3/2
  Demux3/1 -> Mux3/1
  Mux3/1 -> Gain/1
  X_drone/1 -> Tether Dynamics/1(X_drone)
  Tether Dynamics/1(F_tether) -> Sum/4, Demux3/1
  Tether Dynamics/2(M_tether) -> Mux3/3
  Tether Dynamics/3(F_tether_r) -> F_tether_r/1
  Gain/1 -> FM_tether_rxn/1

== system Drone_BBall_Developer/Drone 1 Dynamics/Quadcopter Plant ==
  note: Just enough noise to make
      | the simulation play out a
      | little differently each time
  FM_ext : Inport
  T_L_d : Inport  Port=2
  T_R_d : Inport  Port=3
  Band-Limited White Noise : simulink/Sources/Band-Limited White Noise  Cov=[0.1^2]  Ts=0.1  seed=round(sum(clock))
  Band-Limited White Noise1 : simulink/Sources/Band-Limited White Noise  Cov=[0.1^2]  Ts=0.1  seed=round(sum(clock))+1
  Band-Limited White Noise2 : simulink/Sources/Band-Limited White Noise  Cov=[0.1^2]  Ts=0.1  seed=round(sum(clock))+2
  Ceiling Reactions : Subsystem
  Constant1 : Constant  Value=[0;-m*g]
  Demux : Demux  Outputs=3
  Demux1 : Demux  Outputs=2
  Demux2 : Demux  Outputs=2
  Ground Reactions : Subsystem
  Left Wall Reactions : Subsystem
  Linear Dynamics : Subsystem
  Mux : Mux  Inputs=2
  Mux1 : Mux  Inputs=6
  Mux2 : Mux  Inputs=2
  Mux3 : Mux  Inputs=3
  Right Wall Reactions : Subsystem
  Rotational Dynamics : Subsystem
  Sum : Sum  Inputs=|++
  Sum2 : Sum  Inputs=+|+
  Sum3 : Sum  Inputs=+|+||+|+|+|+
  Thrust Dynamics : Subsystem
  Thrust Dynamics L : Subsystem
  Thrust Resultants : Subsystem
  X_drone : Outport  VectorParamsAs1DForOutWhenUnconnected=off
  T : Outport  Port=2  VectorParamsAs1DForOutWhenUnconnected=off
  wires:
  T_R_d/1 -> Thrust Dynamics/1(T_d)
  T_L_d/1 -> Thrust Dynamics L/1(T_d)
  Thrust Dynamics L/1(T) -> Thrust Resultants/1(T_L), Mux/1
  Thrust Dynamics/1(T) -> Thrust Resultants/2(T_R), Mux/2
  Rotational Dynamics/2(theta_dot) -> Mux1/6  "theta_dot"
  Rotational Dynamics/1(theta) -> Thrust Resultants/3(Theta), Mux1/5  "theta"
  Demux2/1 -> Mux1/2  "x_dot"
  Demux1/2 -> Mux1/3  "y"
  Demux1/1 -> Mux1/1  "x"
  Linear Dynamics/2(p_dot) -> Demux2/1
  Demux2/2 -> Mux1/4  "y_dot"
  Linear Dynamics/1(p) -> Demux1/1
  Mux1/1 -> Ground Reactions/1(X), Left Wall Reactions/1(X), Right Wall Reactions/1(X), Ceiling Reactions/1(X), X_drone/1
  Sum2/1 -> Linear Dynamics/1(F)
  Demux/3 -> Rotational Dynamics/1(M)  "M"
  Mux2/1 -> Sum2/2
  Demux/1 -> Mux2/1  "Fx"
  Demux/2 -> Mux2/2  "Fy"
  Sum3/1 -> Sum/1
  Constant1/1 -> Sum2/1
  Ground Reactions/1(FM_R) -> Sum3/3
  Thrust Resultants/1("FM ") -> Sum3/2
  FM_ext/1 -> Sum3/1
  Mux/1 -> T/1
  Band-Limited White Noise2/1 -> Mux3/3
  Band-Limited White Noise1/1 -> Mux3/2
  Band-Limited White Noise/1 -> Mux3/1
  Sum/1 -> Demux/1
  Mux3/1 -> Sum/2
  Left Wall Reactions/1(FM_R) -> Sum3/4
  Ceiling Reactions/1(FM_R) -> Sum3/6
  Right Wall Reactions/1(FM_R) -> Sum3/5

== system Drone_BBall_Developer/Drone 2 Dynamics/Hook Plant ==
  mag_on : Inport
  X_ball : Inport  Port=2
  X_drone : Inport  Port=3
  Constant : Constant  Value=0
  Constant1 : Constant  Value=[0; -m_hook*g]
  Demux{,1..3} (4 alike) : Demux  Outputs=2
  Ground Reactions : Subsystem
  Hook Dynamics : Subsystem
  Linear Dynamics : Subsystem
  Mux : Mux  Inputs=3
  Mux1 : Mux  Inputs=6
  Mux3 : Mux  Inputs=3
  Sum : Sum  Inputs=+|+-+
  Tether Dynamics : Subsystem
  X_hook : Outport  VectorParamsAs1DForOutWhenUnconnected=off
  FM_ball : Outport  Port=2  VectorParamsAs1DForOutWhenUnconnected=off
  F_tether_r : Outport  Port=3  VectorParamsAs1DForOutWhenUnconnected=off
  FM_tether : Outport  Port=4  VectorParamsAs1DForOutWhenUnconnected=off
  wires:
  Constant/1 -> Mux1/6, Mux1/5
  Demux2/1 -> Mux1/2  "x_dot"
  Demux1/2 -> Mux1/3  "y"
  Demux1/1 -> Mux1/1  "x"
  Linear Dynamics/2(p_dot) -> Demux2/1  "p_dot"
  Demux2/2 -> Mux1/4  "y_dot"
  Linear Dynamics/1(p) -> Demux1/1  "p"
  Constant1/1 -> Sum/1
  Ground Reactions/1(F_R) -> Sum/2
  Sum/1 -> Linear Dynamics/1(F)
  mag_on/1 -> Hook Dynamics/3(mag_on)
  Mux1/1 -> X_hook/1, Ground Reactions/1(X), Tether Dynamics/2(X_hook), Hook Dynamics/1(X_hook)
  X_ball/1 -> Hook Dynamics/2(X_ball)
  Hook Dynamics/1(F_ball) -> Sum/3, Demux/1
  Hook Dynamics/2(M_ball) -> Mux/3
  Mux/1 -> FM_ball/1
  Demux/1 -> Mux/1
  Demux/2 -> Mux/2
  Demux3/2 -> Mux3/2
  Demux3/1 -> Mux3/1
  Mux3/1 -> FM_tether/1
  X_drone/1 -> Tether Dynamics/1(X_drone)
  Tether Dynamics/1(F_tether) -> Sum/4, Demux3/1
  Tether Dynamics/2(M_tether) -> Mux3/3
  Tether Dynamics/3(F_tether_r) -> F_tether_r/1

== system Drone_BBall_Developer/Drone 2 Dynamics/Quadcopter Plant ==
  FM_ext : Inport
  T_L_d : Inport  Port=2
  T_R_d : Inport  Port=3
  Band-Limited White Noise : simulink/Sources/Band-Limited White Noise  Cov=[0.1^2]  Ts=0.1  seed=round(sum(clock))+3
  Band-Limited White Noise1 : simulink/Sources/Band-Limited White Noise  Cov=[0.1^2]  Ts=0.1  seed=round(sum(clock))+4
  Band-Limited White Noise2 : simulink/Sources/Band-Limited White Noise  Cov=[0.1^2]  Ts=0.1  seed=round(sum(clock))+5
  Ceiling Reactions : Subsystem
  Constant1 : Constant  Value=[0;-m*g]
  Demux : Demux  Outputs=3
  Demux1 : Demux  Outputs=2
  Demux2 : Demux  Outputs=2
  Ground Reactions : Subsystem
  Left Wall Reactions : Subsystem
  Linear Dynamics : Subsystem
  Mux : Mux  Inputs=2
  Mux1 : Mux  Inputs=6
  Mux2 : Mux  Inputs=2
  Mux3 : Mux  Inputs=3
  Right Wall Reactions : Subsystem
  Rotational Dynamics : Subsystem
  Sum : Sum  Inputs=|++
  Sum2 : Sum  Inputs=+|+
  Sum3 : Sum  Inputs=+|+||+|+|+|+
  Thrust Dynamics : Subsystem
  Thrust Dynamics L : Subsystem
  Thrust Resultants : Subsystem
  X_drone : Outport  VectorParamsAs1DForOutWhenUnconnected=off
  T : Outport  Port=2  VectorParamsAs1DForOutWhenUnconnected=off
  wires:
  T_R_d/1 -> Thrust Dynamics/1(T_d)
  T_L_d/1 -> Thrust Dynamics L/1(T_d)
  Thrust Dynamics L/1(T) -> Thrust Resultants/1(T_L), Mux/1
  Thrust Dynamics/1(T) -> Thrust Resultants/2(T_R), Mux/2
  Rotational Dynamics/2(theta_dot) -> Mux1/6  "theta_dot"
  Rotational Dynamics/1(theta) -> Thrust Resultants/3(Theta), Mux1/5  "theta"
  Demux2/1 -> Mux1/2  "x_dot"
  Demux1/2 -> Mux1/3  "y"
  Demux1/1 -> Mux1/1  "x"
  Linear Dynamics/2(p_dot) -> Demux2/1
  Demux2/2 -> Mux1/4  "y_dot"
  Linear Dynamics/1(p) -> Demux1/1
  Mux1/1 -> Ground Reactions/1(X), Left Wall Reactions/1(X), Right Wall Reactions/1(X), Ceiling Reactions/1(X), X_drone/1
  Sum2/1 -> Linear Dynamics/1(F)
  Demux/3 -> Rotational Dynamics/1(M)  "M"
  Mux2/1 -> Sum2/2
  Demux/1 -> Mux2/1  "Fx"
  Demux/2 -> Mux2/2  "Fy"
  Sum3/1 -> Sum/1
  Constant1/1 -> Sum2/1
  Ground Reactions/1(FM_R) -> Sum3/3
  Thrust Resultants/1("FM ") -> Sum3/2
  FM_ext/1 -> Sum3/1
  Mux/1 -> T/1
  Band-Limited White Noise2/1 -> Mux3/3
  Band-Limited White Noise1/1 -> Mux3/2
  Band-Limited White Noise/1 -> Mux3/1
  Sum/1 -> Demux/1
  Mux3/1 -> Sum/2
  Left Wall Reactions/1(FM_R) -> Sum3/4
  Ceiling Reactions/1(FM_R) -> Sum3/6
  Right Wall Reactions/1(FM_R) -> Sum3/5

== system Drone_BBall_Developer/EMP Mechanics//Dynamics/Drone-EMP Collision 1 ==
  X_emp : Inport
  X_drone : Inport  Port=2
  Constant4 : Constant  Value=r
  Demux : Demux  Outputs=2
  Less Than : RelationalOperator  Operator=<  OutDataTypeStr=boolean  RndMeth=Simplest
  Mux : Mux  Inputs=2
  Norm : Fcn  Expr=sqrt(u(1)^2+u(2)^2)+1e-10
  Selector : Selector  InputPortWidth=6  IndexOptions=Index vector (dialog)  Indices=[1 3]  OutputSizes=1
  Sum : Sum  Inputs=+-
  Collision : Outport  VectorParamsAs1DForOutWhenUnconnected=off
  wires:
  X_drone/1 -> Sum/1
  X_emp/1 -> Sum/2
  Sum/1 -> Selector/1
  Less Than/1 -> Collision/1
  Norm/1 -> Less Than/1  "distance"
  Constant4/1 -> Less Than/2
  Selector/1 -> Demux/1
  Demux/2 -> Mux/2
  Demux/1 -> Mux/1
  Mux/1 -> Norm/1

== system Drone_BBall_Developer/EMP Mechanics//Dynamics/Drone-EMP Collision 2 ==
  X_emp : Inport
  X_drone : Inport  Port=2
  Constant4 : Constant  Value=r
  Demux : Demux  Outputs=2
  Less Than : RelationalOperator  Operator=<  OutDataTypeStr=boolean  RndMeth=Simplest
  Mux : Mux  Inputs=2
  Norm : Fcn  Expr=sqrt(u(1)^2+u(2)^2)+1e-10
  Selector : Selector  InputPortWidth=6  IndexOptions=Index vector (dialog)  Indices=[1 3]  OutputSizes=1
  Sum : Sum  Inputs=+-
  Collision : Outport  VectorParamsAs1DForOutWhenUnconnected=off
  wires:
  X_drone/1 -> Sum/1
  X_emp/1 -> Sum/2
  Sum/1 -> Selector/1
  Selector/1 -> Demux/1
  Less Than/1 -> Collision/1
  Norm/1 -> Less Than/1  "distance"
  Constant4/1 -> Less Than/2
  Demux/2 -> Mux/2
  Demux/1 -> Mux/1
  Mux/1 -> Norm/1

== system Drone_BBall_Developer/EMP Mechanics//Dynamics/Drone-EMP Logic 1 ==
  Fire EMP : Inport
  EMP Hit : Inport  Port=2
  Drone Hit : Inport  Port=3
  AND : Logic  Inputs=3  AllPortsSameDT=off  OutDataTypeStr=boolean
  AND1 : Logic  Operator=OR  AllPortsSameDT=off  OutDataTypeStr=boolean
  AND2 : Logic  AllPortsSameDT=off  OutDataTypeStr=boolean
  AND3 : Logic  Operator=OR  AllPortsSameDT=off  OutDataTypeStr=boolean
  AND4 : Logic  AllPortsSameDT=off  OutDataTypeStr=boolean
  Detect EMP Release : dspswit3/Edge Detector
      settings: SourceProductBaseCode=DS
  Gain : Gain
  Memory : Memory
  Memory1 : Memory
  Memory2 : Memory
  NOT{1..4} (4 alike) : Logic  Operator=NOT  IconShape=distinctive  AllPortsSameDT=off  OutDataTypeStr=boolean
  Recharge Timer : dspswit3/Counter  Direction=Up  CountEvent=Free running  CounterSize=User defined  MaxCount=1e10  InitialCount=0  Output=Hit  HitValue=2000  ResetInput=on  SamplesPerFrame=1  Ts=.001  CntDtype=double  HitDtype=Logical
  Rst to 0 = armed Inc to 1 = not armed : dspswit3/Counter  Direction=Up  CountEvent=Rising edge  CounterSize=User defined  MaxCount=1e10  InitialCount=0  Output=Count  HitValue=1  ResetInput=on  SamplesPerFrame=1  Ts=.1  CntDtype=double  HitDtype=Logical
  Rst to 0 = not stunned Inc to 1 = stunned : dspswit3/Counter  Direction=Up  CountEvent=Rising edge  CounterSize=User defined  MaxCount=1e10  InitialCount=0  Output=Count  HitValue=1  ResetInput=on  SamplesPerFrame=1  Ts=.1  CntDtype=double  HitDtype=Logical
  Rst to 0 = visible Inc to 1 = not visible : dspswit3/Counter  Direction=Up  CountEvent=Rising edge  CounterSize=User defined  MaxCount=1e10  InitialCount=0  Output=Count  HitValue=1  ResetInput=on  SamplesPerFrame=1  Ts=.1  CntDtype=double  HitDtype=Logical
  Stun Timer : dspswit3/Counter  Direction=Up  CountEvent=Free running  CounterSize=User defined  MaxCount=1e10  InitialCount=0  Output=Hit  HitValue=1000  ResetInput=on  SamplesPerFrame=1  Ts=.001  CntDtype=double  HitDtype=Logical
  Stunned : Outport  VectorParamsAs1DForOutWhenUnconnected=off
  EMP Visible : Outport  Port=2  VectorParamsAs1DForOutWhenUnconnected=off
  EMP Armed : Outport  Port=3  VectorParamsAs1DForOutWhenUnconnected=off
  EMP Live : Outport  Port=4  VectorParamsAs1DForOutWhenUnconnected=off
  Reset EMP : Outport  Port=5  VectorParamsAs1DForOutWhenUnconnected=off
  wires:
  Recharge Timer/1 -> Rst to 0 = visible Inc to 1 = not visible/2, Rst to 0 = armed Inc to 1 = not armed/2
  AND/1 -> AND1/1
  Memory/1 -> NOT3/1, AND1/2  "not armed"
  Fire EMP/1 -> AND/2
  NOT3/1 -> EMP Armed/1, AND/3  "armed"
  AND1/1 -> AND2/2, NOT2/1, Detect EMP Release/1  "let fly"
  Rst to 0 = armed Inc to 1 = not armed/1 -> Memory/1
  NOT2/1 -> Reset EMP/1
  Detect EMP Release/1 -> Rst to 0 = armed Inc to 1 = not armed/1, Recharge Timer/1
  EMP Hit/1 -> Rst to 0 = visible Inc to 1 = not visible/1
  AND2/1 -> EMP Live/1, AND3/2
  Rst to 0 = visible Inc to 1 = not visible/1 -> Memory1/1
  Memory1/1 -> NOT1/1  "not visible"
  NOT1/1 -> AND4/2, AND2/1  "visible"
  Stun Timer/1 -> Rst to 0 = not stunned Inc to 1 = stunned/2
  Memory2/1 -> NOT4/1, Stunned/1  "stunned"
  Rst to 0 = not stunned Inc to 1 = stunned/1 -> Memory2/1
  Drone Hit/1 -> Rst to 0 = not stunned Inc to 1 = stunned/1, Stun Timer/1
  Gain/1 -> EMP Visible/1
  NOT4/1 -> AND3/1, AND/1
  AND3/1 -> AND4/1
  AND4/1 -> Gain/1

== system Drone_BBall_Developer/EMP Mechanics//Dynamics/Drone-EMP Logic 2 ==
  Fire EMP : Inport
  EMP Hit : Inport  Port=2
  Drone Hit : Inport  Port=3
  AND : Logic  Inputs=3  AllPortsSameDT=off  OutDataTypeStr=boolean
  AND1 : Logic  Operator=OR  AllPortsSameDT=off  OutDataTypeStr=boolean
  AND2 : Logic  AllPortsSameDT=off  OutDataTypeStr=boolean
  AND3 : Logic  Operator=OR  AllPortsSameDT=off  OutDataTypeStr=boolean
  AND4 : Logic  AllPortsSameDT=off  OutDataTypeStr=boolean
  Detect EMP Release : dspswit3/Edge Detector
      settings: SourceProductBaseCode=DS
  Gain : Gain
  Memory : Memory
  Memory1 : Memory
  Memory2 : Memory
  NOT{1..4} (4 alike) : Logic  Operator=NOT  IconShape=distinctive  AllPortsSameDT=off  OutDataTypeStr=boolean
  Recharge Timer : dspswit3/Counter  Direction=Up  CountEvent=Free running  CounterSize=User defined  MaxCount=1e10  InitialCount=0  Output=Hit  HitValue=2000  ResetInput=on  SamplesPerFrame=1  Ts=.001  CntDtype=double  HitDtype=Logical
  Rst to 0 = armed Inc to 1 = not armed : dspswit3/Counter  Direction=Up  CountEvent=Rising edge  CounterSize=User defined  MaxCount=1e10  InitialCount=0  Output=Count  HitValue=1  ResetInput=on  SamplesPerFrame=1  Ts=.1  CntDtype=double  HitDtype=Logical
  Rst to 0 = not stunned Inc to 1 = stunned : dspswit3/Counter  Direction=Up  CountEvent=Rising edge  CounterSize=User defined  MaxCount=1e10  InitialCount=0  Output=Count  HitValue=1  ResetInput=on  SamplesPerFrame=1  Ts=.1  CntDtype=double  HitDtype=Logical
  Rst to 0 = visible Inc to 1 = not visible : dspswit3/Counter  Direction=Up  CountEvent=Rising edge  CounterSize=User defined  MaxCount=1e10  InitialCount=0  Output=Count  HitValue=1  ResetInput=on  SamplesPerFrame=1  Ts=.1  CntDtype=double  HitDtype=Logical
  Stun Timer : dspswit3/Counter  Direction=Up  CountEvent=Free running  CounterSize=User defined  MaxCount=1e10  InitialCount=0  Output=Hit  HitValue=1000  ResetInput=on  SamplesPerFrame=1  Ts=.001  CntDtype=double  HitDtype=Logical
  Stunned : Outport  VectorParamsAs1DForOutWhenUnconnected=off
  EMP Visible : Outport  Port=2  VectorParamsAs1DForOutWhenUnconnected=off
  EMP Armed : Outport  Port=3  VectorParamsAs1DForOutWhenUnconnected=off
  EMP Live : Outport  Port=4  VectorParamsAs1DForOutWhenUnconnected=off
  Reset EMP : Outport  Port=5  VectorParamsAs1DForOutWhenUnconnected=off
  wires:
  Recharge Timer/1 -> Rst to 0 = visible Inc to 1 = not visible/2, Rst to 0 = armed Inc to 1 = not armed/2
  AND/1 -> AND1/1
  Memory/1 -> NOT3/1, AND1/2  "not armed"
  Fire EMP/1 -> AND/2
  NOT3/1 -> EMP Armed/1, AND/3  "armed"
  AND1/1 -> AND2/2, NOT2/1, Detect EMP Release/1  "let fly"
  Rst to 0 = armed Inc to 1 = not armed/1 -> Memory/1
  NOT2/1 -> Reset EMP/1
  Detect EMP Release/1 -> Rst to 0 = armed Inc to 1 = not armed/1, Recharge Timer/1
  EMP Hit/1 -> Rst to 0 = visible Inc to 1 = not visible/1
  AND2/1 -> EMP Live/1, AND3/2
  Rst to 0 = visible Inc to 1 = not visible/1 -> Memory1/1
  Memory1/1 -> NOT1/1  "not visible"
  NOT1/1 -> AND4/2, AND2/1  "visible"
  Stun Timer/1 -> Rst to 0 = not stunned Inc to 1 = stunned/2
  Memory2/1 -> NOT4/1, Stunned/1  "stunned"
  Rst to 0 = not stunned Inc to 1 = stunned/1 -> Memory2/1
  Drone Hit/1 -> Rst to 0 = not stunned Inc to 1 = stunned/1, Stun Timer/1
  Gain/1 -> EMP Visible/1
  NOT4/1 -> AND3/1, AND/1
  AND3/1 -> AND4/1
  AND4/1 -> Gain/1
